simulink model "MRC_regulator"  (R2021b)
settings: Solver=VariableStepAuto  StartTime=0.0  StopTime=100  RelTol=1e-3
undefined symbols (not defined in the file): a0, am, b0, bm, input, pGain, pT, theta1_ideal, theta2_ideal, upb
settings Model: Creator=miso  LastModifiedBy=user

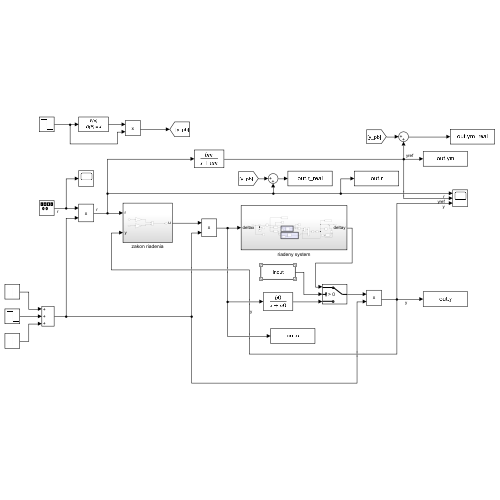
[thumbnail: Simulink's stored preview of the top-level diagram]
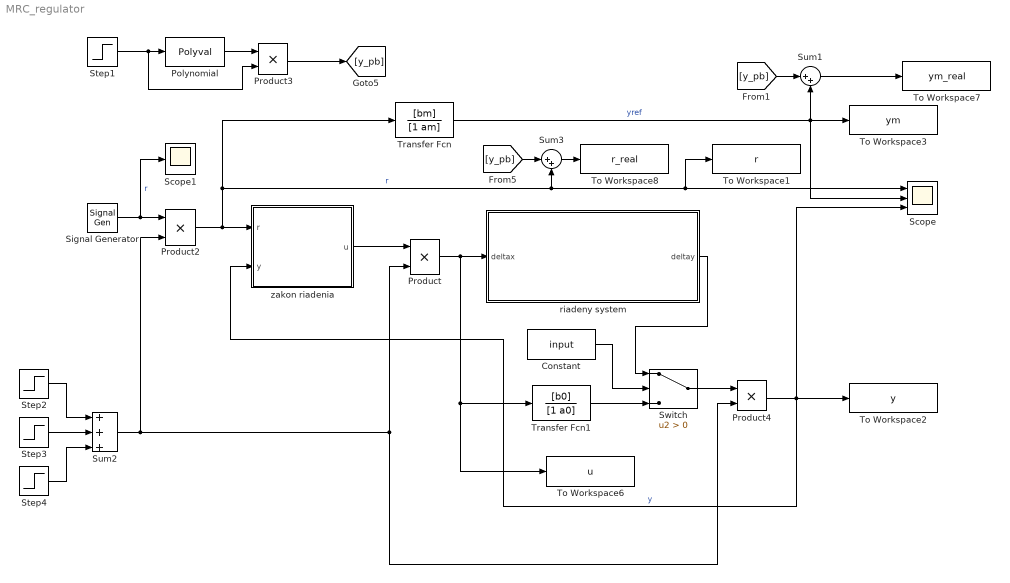
== system MRC_regulator ==
  Constant : Constant  Value=input
  Polynomial : Polyval  Coefs=pGain
  Product{,2..4} (4 alike) : Product
  Scope : Scope  NumInputPorts=3
  Scope1 : Scope
  Signal Generator : SignalGenerator  WaveForm=square  Amplitude=-6  Frequency=1/10
  Step1 : Step  Time=50  Before=upb  After=upb-upb_delta  SampleTime=0
  Step2 : Step  Time=10  SampleTime=0
  Step3 : Step  Time=45  Before=1  After=0  SampleTime=0
  Step4 : Step  Time=60  Before=-1  After=0  SampleTime=0
  Sum1 : Sum  Inputs=|++
  Sum2 : Sum  Inputs=+++
  Sum3 : Sum  Inputs=|++
  Switch : Switch  Criteria=u2 > Threshold
  To Workspace1 : ToWorkspace  VariableName=r  SaveFormat=Timeseries  SampleTime=-1
  To Workspace2 : ToWorkspace  VariableName=y  SaveFormat=Timeseries  SampleTime=-1
  To Workspace3 : ToWorkspace  VariableName=ym  SaveFormat=Timeseries  SampleTime=-1
  To Workspace6 : ToWorkspace  VariableName=u  SaveFormat=Timeseries  SampleTime=-1
  To Workspace7 : ToWorkspace  VariableName=ym_real  SaveFormat=Timeseries  SampleTime=-1
  To Workspace8 : ToWorkspace  VariableName=r_real  SaveFormat=Timeseries  SampleTime=-1
  Transfer Fcn : TransferFcn  Numerator=[bm]  Denominator=[1 am]
  Transfer Fcn1 : TransferFcn  Numerator=[b0]  Denominator=[1 a0]
  riadeny system : Subsystem
  zakon riadenia : Subsystem
  wires:
  Product/1 -> riadeny system/1(deltax), Transfer Fcn1/1, To Workspace6/1
  Sum2/1 -> Product2/2, Product4/2, Product/2
  Product2/1 -> Transfer Fcn/1, To Workspace1/1, Scope/1, Sum3/2, zakon riadenia/1(r)  "r"
  zakon riadenia/1(u) -> Product/1
  Product4/1 -> To Workspace2/1, Scope/3, zakon riadenia/2(y)  "y"
  Switch/1 -> Product4/1
  Signal Generator/1 -> Scope1/1, Product2/1  "r"
  Sum3/1 -> To Workspace8/1
  Step1/1 -> Product3/2, Polynomial/1
  [y_pb] -> Sum3/1
  Product3/1 -> [y_pb]
  Polynomial/1 -> Product3/1
  [y_pb] -> Sum1/1
  Transfer Fcn/1 -> To Workspace3/1, Scope/2, Sum1/2  "yref"
  Sum1/1 -> To Workspace7/1
  Step3/1 -> Sum2/2
  Step2/1 -> Sum2/1
  Step4/1 -> Sum2/3
  Constant/1 -> Switch/2
  riadeny system/1(deltay) -> Switch/1
  Transfer Fcn1/1 -> Switch/3

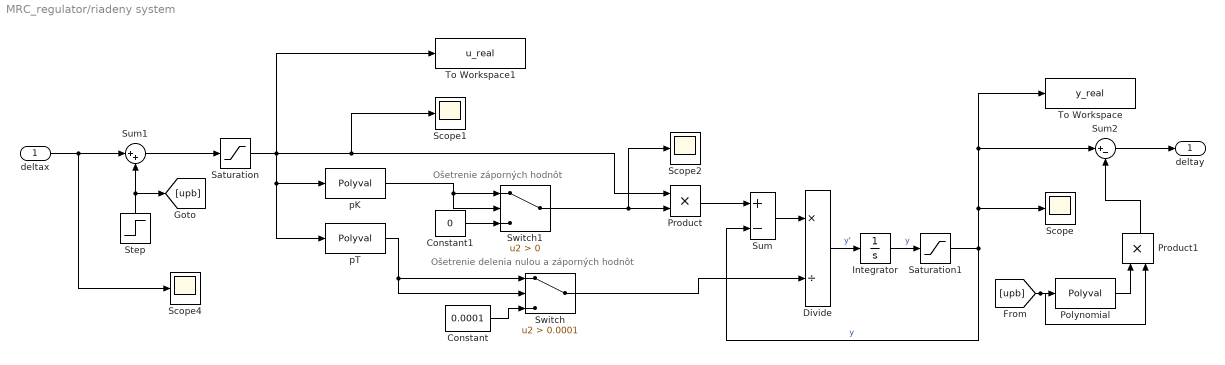
== system MRC_regulator/riadeny system ==
  note: Ošetrenie delenia nulou a záporných hodnôt
  note: Ošetrenie záporných hodnôt
  deltax : Inport
  Constant : Constant  Value=0.0001
  Constant1 : Constant  Value=0
  Divide : Product  Inputs=*/
  Integrator : Integrator
  Polynomial : Polyval  Coefs=pGain
  Product : Product
  Product1 : Product
  Saturation : Saturate  UpperLimit=255  LowerLimit=0
  Saturation1 : Saturate  UpperLimit=1023  LowerLimit=0
  Scope{,1..2,4} (4 alike) : Scope
  Step : Step  Time=50  Before=upb  After=upb-upb_delta  SampleTime=0
  Sum : Sum  Inputs=+-
  Sum1 : Sum  Inputs=|++
  Sum2 : Sum  Inputs=|+-
  Switch : Switch  Criteria=u2 > Threshold  Threshold=0.0001
  Switch1 : Switch  Criteria=u2 > Threshold
  To Workspace : ToWorkspace  VariableName=y_real  SaveFormat=Timeseries  SampleTime=-1
  To Workspace1 : ToWorkspace  VariableName=u_real  SaveFormat=Timeseries  SampleTime=-1
  pK : Polyval  Coefs=pGain
  pT : Polyval  Coefs=pT
  deltay : Outport
  wires:
  Sum/1 -> Divide/1
  Saturation1/1 -> To Workspace/1, Sum2/1, Scope/1, Sum/2  "y"
  Constant/1 -> Switch/3
  pT/1 -> Switch/1, Switch/2
  pK/1 -> Switch1/2, Switch1/1
  Switch/1 -> Divide/2
  Constant1/1 -> Switch1/3
  Product/1 -> Sum/1
  Switch1/1 -> Scope2/1, Product/2
  Integrator/1 -> Saturation1/1  "y"
  Divide/1 -> Integrator/1  "y'"
  deltax/1 -> Scope4/1, Sum1/1
  Sum1/1 -> Saturation/1
  Saturation/1 -> To Workspace1/1, pT/1, pK/1, Scope1/1, Product/1
  Sum2/1 -> deltay/1
  Polynomial/1 -> Product1/1
  Step/1 -> [upb], Sum1/2
  [upb] -> Product1/2, Polynomial/1
  Product1/1 -> Sum2/2

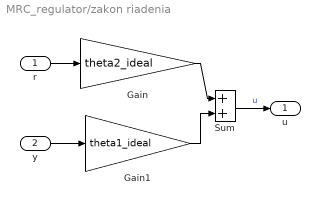
== system MRC_regulator/zakon riadenia ==
  r : Inport
  y : Inport  Port=2
  Gain : Gain  Gain=theta2_ideal
  Gain1 : Gain  Gain=theta1_ideal
  Sum : Sum
  u : Outport
  wires:
  Gain/1 -> Sum/1
  Gain1/1 -> Sum/2
  y/1 -> Gain1/1
  Sum/1 -> u/1  "u"
  r/1 -> Gain/1
